simulink model "Task4"  (R2022a)
settings: Solver=VariableStepAuto  StartTime=0.0  StopTime=25  RelTol=1e-3
settings Model: Creator=Family  LastModifiedBy=Family

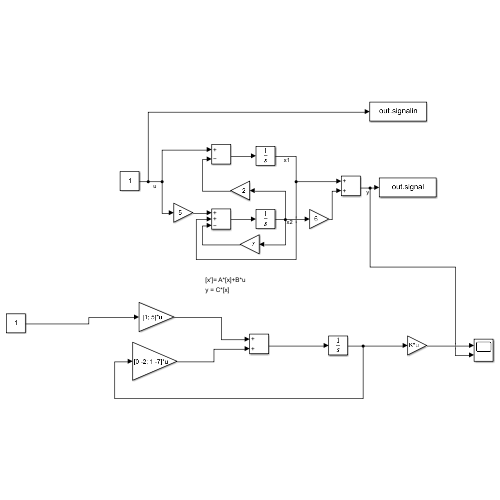
[thumbnail: Simulink's stored preview of the top-level diagram]
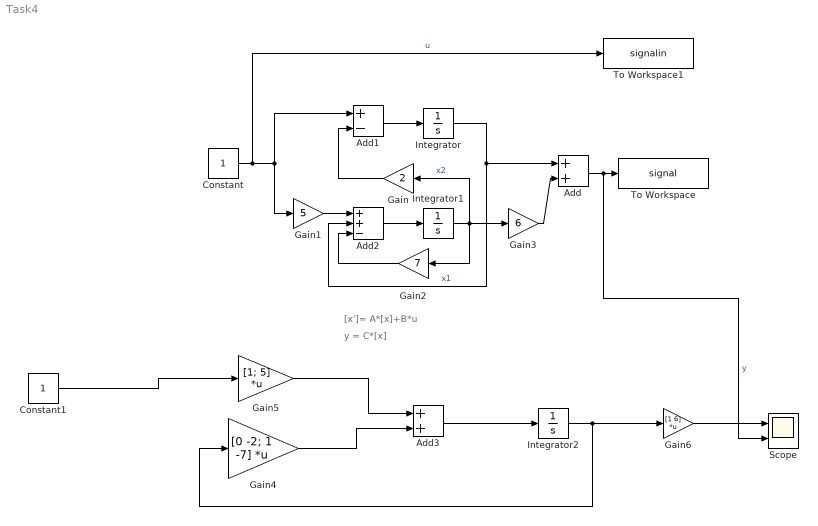
== system Task4 ==
  note: y = C*[x]
  note: [x']= A*[x]+B*u
  Add : Sum
  Add1 : Sum  Inputs=+-
  Add2 : Sum  Inputs=++-
  Add3 : Sum
  Constant : Constant  SampleTime=-1
  Constant1 : Constant  SampleTime=-1
  Gain : Gain  Gain=2
  Gain1 : Gain  Gain=5
  Gain2 : Gain  Gain=7
  Gain3 : Gain  Gain=6
  Gain4 : Gain  Gain=[0 -2; 1 -7]  Multiplication=Matrix(K*u)
  Gain5 : Gain  Gain=[1; 5]  Multiplication=Matrix(K*u)
  Gain6 : Gain  Gain=[1 6]  Multiplication=Matrix(K*u)
  Integrator : Integrator
  Integrator1 : Integrator
  Integrator2 : Integrator
  Scope : Scope  NumInputPorts=2
  To Workspace : ToWorkspace  VariableName=signal  SaveFormat=Timeseries  SampleTime=-1
  To Workspace1 : ToWorkspace  VariableName=signalin  SaveFormat=Timeseries  SampleTime=-1
  wires:
  Add/1 -> Scope/2, To Workspace/1  "y"
  Integrator/1 -> Add2/2, Add/1  "x1"
  Integrator1/1 -> Gain/1, Gain3/1, Gain2/1  "x2"
  Add1/1 -> Integrator/1
  Gain/1 -> Add1/2
  Constant/1 -> To Workspace1/1, Gain1/1, Add1/1  "u"
  Add2/1 -> Integrator1/1
  Gain1/1 -> Add2/1
  Gain2/1 -> Add2/3
  Gain3/1 -> Add/2
  Integrator2/1 -> Gain6/1, Gain4/1
  Gain4/1 -> Add3/2
  Add3/1 -> Integrator2/1
  Constant1/1 -> Gain5/1
  Gain5/1 -> Add3/1
  Gain6/1 -> Scope/1
